simulink model "myproject_task"  (Simulink 3.00)
libraries: mathlib x17, inoutlib x13

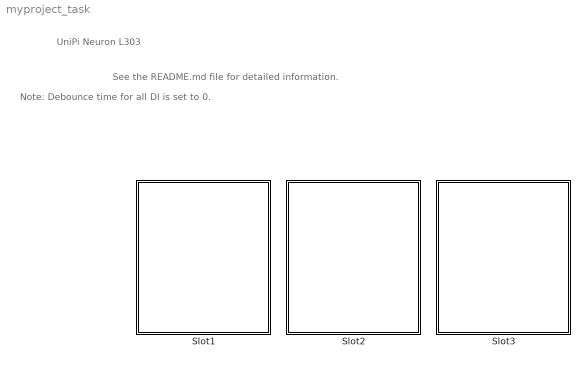
== system myproject_task ==
  note: See the README.md file for detailed information.
  note: UniPi Neuron L303
  note: Note: Debounce time for all DI is set to 0.
  Slot1 : Subsystem
      mask Type: REX sequence
  Slot2 : Subsystem
      mask Type: REX sequence
  Slot3 : Subsystem
      mask Type: REX sequence

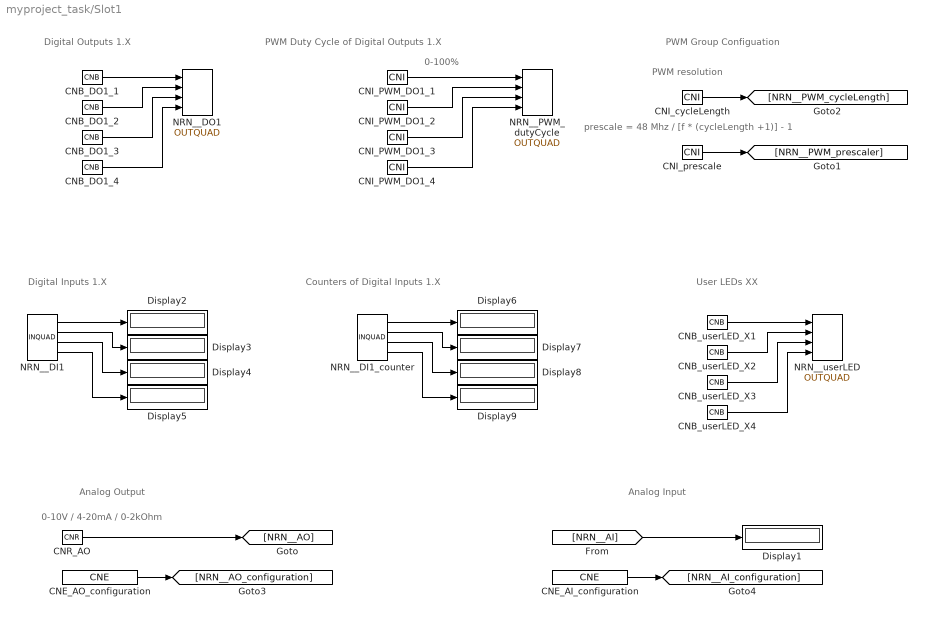
== system myproject_task/Slot1 ==
  note: 0-100%
  note: PWM resolution
  note: prescale = 48 Mhz / [f * (cycleLength +1)] - 1
  note: Digital Inputs 1.X
  note: Counters of Digital Inputs 1.X
  note: Digital Outputs 1.X
  note: User LEDs XX
  note: PWM Duty Cycle of Digital Outputs 1.X
  note: PWM Group Configuation
  note: 0-10V / 4-20mA / 0-2kOhm
  note: Analog Output
  note: Analog Input
  CNB_DO1_{1..4} (4 alike) : mathlib/CNB  YCN=off
  CNB_userLED_X{1..4} (4 alike) : mathlib/CNB  YCN=off
  CNE_AI_configuration : mathlib/CNE  yenum=0: Voltage 0-10V  pupstr=0: Voltage 0-10V|1: Current 0-20mA
  CNE_AO_configuration : mathlib/CNE  yenum=0: Voltage 0-10V  pupstr=0: Voltage 0-10V|1: Current 0-20mA|3: Resistance 0-2kOhm
  CNI_PWM_DO1_{1..4} (4 alike) : mathlib/CNI  icn=0
  CNI_cycleLength : mathlib/CNI  icn=1024
  CNI_prescale : mathlib/CNI  icn=467
  CNR_AO : mathlib/CNR  ycn=0
  Display{1..9} (9 alike) : Display
      Display1 settings: Format=short
      Display2 settings: Format=bin
      Display3 settings: Format=bin
      Display4 settings: Format=bin
      Display5 settings: Format=bin
      Display6 settings: Format=Best fit
      Display7 settings: Format=Best fit
      Display8 settings: Format=Best fit
      Display9 settings: Format=Best fit
  NRN__DI1 : inoutlib/INQUAD
  NRN__DI1_counter : inoutlib/INQUAD
  NRN__DO1 : inoutlib/OUTQUAD
  NRN__PWM_dutyCycle : inoutlib/OUTQUAD
  NRN__userLED : inoutlib/OUTQUAD
  wires:
  CNB_DO1_1/1 -> NRN__DO1/1
  CNB_DO1_2/1 -> NRN__DO1/2
  CNB_DO1_3/1 -> NRN__DO1/3
  CNB_DO1_4/1 -> NRN__DO1/4
  CNB_userLED_X1/1 -> NRN__userLED/1
  CNB_userLED_X2/1 -> NRN__userLED/2
  CNB_userLED_X3/1 -> NRN__userLED/3
  CNB_userLED_X4/1 -> NRN__userLED/4
  CNE_AI_configuration/1 -> [NRN__AI_configuration]
  CNE_AO_configuration/1 -> [NRN__AO_configuration]
  CNI_PWM_DO1_1/1 -> NRN__PWM_dutyCycle/1
  CNI_PWM_DO1_2/1 -> NRN__PWM_dutyCycle/2
  CNI_PWM_DO1_3/1 -> NRN__PWM_dutyCycle/3
  CNI_PWM_DO1_4/1 -> NRN__PWM_dutyCycle/4
  CNI_cycleLength/1 -> [NRN__PWM_cycleLength]
  CNI_prescale/1 -> [NRN__PWM_prescaler]
  CNR_AO/1 -> [NRN__AO]
  [NRN__AI] -> Display1/1
  NRN__DI1/1 -> Display2/1
  NRN__DI1/2 -> Display3/1
  NRN__DI1/3 -> Display4/1
  NRN__DI1/4 -> Display5/1
  NRN__DI1_counter/1 -> Display6/1
  NRN__DI1_counter/2 -> Display7/1
  NRN__DI1_counter/3 -> Display8/1
  NRN__DI1_counter/4 -> Display9/1

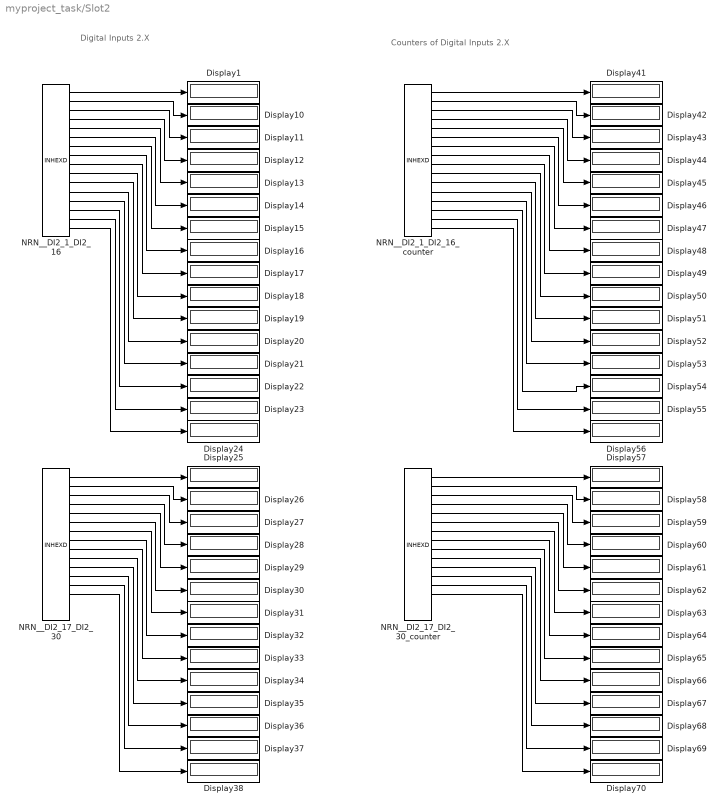
== system myproject_task/Slot2 ==
  note: Digital Inputs 2.X
  note: Counters of Digital Inputs 2.X
  Display{1,10..38,41..70} (60 alike) : Display
      Display1 settings: Format=bin
      Display10 settings: Format=bin
      Display11 settings: Format=bin
      Display12 settings: Format=bin
      Display13 settings: Format=bin
      Display14 settings: Format=bin
      Display15 settings: Format=bin
      Display16 settings: Format=bin
      Display17 settings: Format=bin
      Display18 settings: Format=bin
      Display19 settings: Format=bin
      Display20 settings: Format=bin
      Display21 settings: Format=bin
      Display22 settings: Format=bin
      Display23 settings: Format=bin
      Display24 settings: Format=bin
      Display25 settings: Format=bin
      Display26 settings: Format=bin
      Display27 settings: Format=bin
      Display28 settings: Format=bin
      Display29 settings: Format=bin
      Display30 settings: Format=bin
      Display31 settings: Format=bin
      Display32 settings: Format=bin
      Display33 settings: Format=bin
      Display34 settings: Format=bin
      Display35 settings: Format=bin
      Display36 settings: Format=bin
      Display37 settings: Format=bin
      Display38 settings: Format=bin
      Display41 settings: Format=Best fit
      Display42 settings: Format=Best fit
      Display43 settings: Format=Best fit
      Display44 settings: Format=Best fit
      Display45 settings: Format=Best fit
      Display46 settings: Format=Best fit
      Display47 settings: Format=Best fit
      Display48 settings: Format=Best fit
      Display49 settings: Format=Best fit
      Display50 settings: Format=Best fit
      Display51 settings: Format=Best fit
      Display52 settings: Format=Best fit
      Display53 settings: Format=Best fit
      Display54 settings: Format=Best fit
      Display55 settings: Format=Best fit
      Display56 settings: Format=Best fit
      Display57 settings: Format=Best fit
      Display58 settings: Format=Best fit
      Display59 settings: Format=Best fit
      Display60 settings: Format=Best fit
      Display61 settings: Format=Best fit
      Display62 settings: Format=Best fit
      Display63 settings: Format=Best fit
      Display64 settings: Format=Best fit
      Display65 settings: Format=Best fit
      Display66 settings: Format=Best fit
      Display67 settings: Format=Best fit
      Display68 settings: Format=Best fit
      Display69 settings: Format=Best fit
      Display70 settings: Format=Best fit
  NRN__DI2_17_DI2_30 : inoutlib/INHEXD
  NRN__DI2_17_DI2_30_counter : inoutlib/INHEXD
  NRN__DI2_1_DI2_16 : inoutlib/INHEXD
  NRN__DI2_1_DI2_16_counter : inoutlib/INHEXD
  wires:
  NRN__DI2_17_DI2_30/1 -> Display25/1
  NRN__DI2_17_DI2_30/2 -> Display26/1
  NRN__DI2_17_DI2_30/3 -> Display27/1
  NRN__DI2_17_DI2_30/4 -> Display28/1
  NRN__DI2_17_DI2_30/5 -> Display29/1
  NRN__DI2_17_DI2_30/6 -> Display30/1
  NRN__DI2_17_DI2_30/7 -> Display31/1
  NRN__DI2_17_DI2_30/8 -> Display32/1
  NRN__DI2_17_DI2_30/9 -> Display33/1
  NRN__DI2_17_DI2_30/10 -> Display34/1
  NRN__DI2_17_DI2_30/11 -> Display35/1
  NRN__DI2_17_DI2_30/12 -> Display36/1
  NRN__DI2_17_DI2_30/13 -> Display37/1
  NRN__DI2_17_DI2_30/14 -> Display38/1
  NRN__DI2_17_DI2_30_counter/1 -> Display57/1
  NRN__DI2_17_DI2_30_counter/2 -> Display58/1
  NRN__DI2_17_DI2_30_counter/3 -> Display59/1
  NRN__DI2_17_DI2_30_counter/4 -> Display60/1
  NRN__DI2_17_DI2_30_counter/5 -> Display61/1
  NRN__DI2_17_DI2_30_counter/6 -> Display62/1
  NRN__DI2_17_DI2_30_counter/7 -> Display63/1
  NRN__DI2_17_DI2_30_counter/8 -> Display64/1
  NRN__DI2_17_DI2_30_counter/9 -> Display65/1
  NRN__DI2_17_DI2_30_counter/10 -> Display66/1
  NRN__DI2_17_DI2_30_counter/11 -> Display67/1
  NRN__DI2_17_DI2_30_counter/12 -> Display68/1
  NRN__DI2_17_DI2_30_counter/13 -> Display69/1
  NRN__DI2_17_DI2_30_counter/14 -> Display70/1
  NRN__DI2_1_DI2_16/1 -> Display1/1
  NRN__DI2_1_DI2_16/2 -> Display10/1
  NRN__DI2_1_DI2_16/3 -> Display11/1
  NRN__DI2_1_DI2_16/4 -> Display12/1
  NRN__DI2_1_DI2_16/5 -> Display13/1
  NRN__DI2_1_DI2_16/6 -> Display14/1
  NRN__DI2_1_DI2_16/7 -> Display15/1
  NRN__DI2_1_DI2_16/8 -> Display16/1
  NRN__DI2_1_DI2_16/9 -> Display17/1
  NRN__DI2_1_DI2_16/10 -> Display18/1
  NRN__DI2_1_DI2_16/11 -> Display19/1
  NRN__DI2_1_DI2_16/12 -> Display20/1
  NRN__DI2_1_DI2_16/13 -> Display21/1
  NRN__DI2_1_DI2_16/14 -> Display22/1
  NRN__DI2_1_DI2_16/15 -> Display23/1
  NRN__DI2_1_DI2_16/16 -> Display24/1
  NRN__DI2_1_DI2_16_counter/1 -> Display41/1
  NRN__DI2_1_DI2_16_counter/2 -> Display42/1
  NRN__DI2_1_DI2_16_counter/3 -> Display43/1
  NRN__DI2_1_DI2_16_counter/4 -> Display44/1
  NRN__DI2_1_DI2_16_counter/5 -> Display45/1
  NRN__DI2_1_DI2_16_counter/6 -> Display46/1
  NRN__DI2_1_DI2_16_counter/7 -> Display47/1
  NRN__DI2_1_DI2_16_counter/8 -> Display48/1
  NRN__DI2_1_DI2_16_counter/9 -> Display49/1
  NRN__DI2_1_DI2_16_counter/10 -> Display50/1
  NRN__DI2_1_DI2_16_counter/11 -> Display51/1
  NRN__DI2_1_DI2_16_counter/12 -> Display52/1
  NRN__DI2_1_DI2_16_counter/13 -> Display53/1
  NRN__DI2_1_DI2_16_counter/14 -> Display54/1
  NRN__DI2_1_DI2_16_counter/15 -> Display55/1
  NRN__DI2_1_DI2_16_counter/16 -> Display56/1

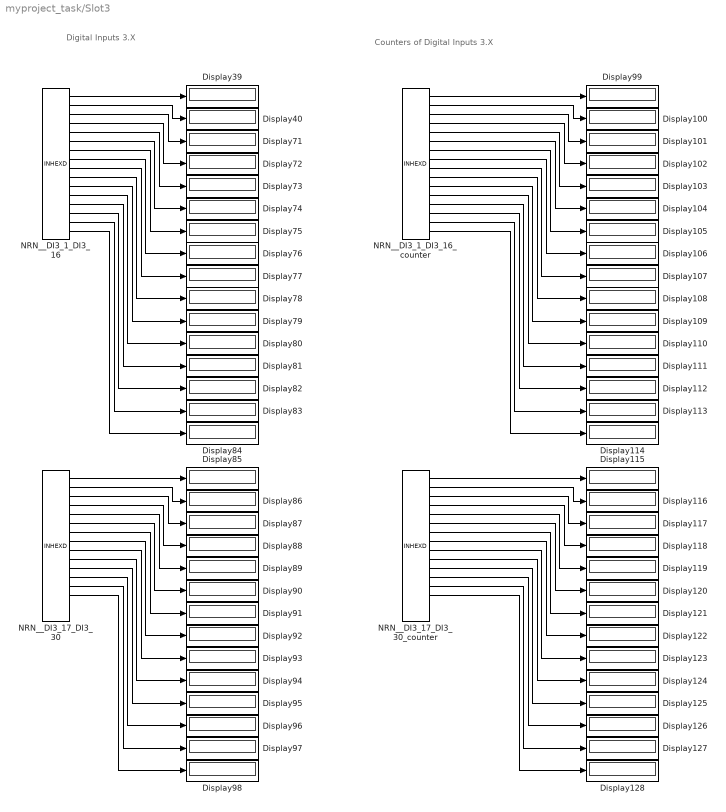
== system myproject_task/Slot3 ==
  note: Digital Inputs 3.X
  note: Counters of Digital Inputs 3.X
  Display{39..40,71..128} (60 alike) : Display
      Display100 settings: Format=Best fit
      Display101 settings: Format=Best fit
      Display102 settings: Format=Best fit
      Display103 settings: Format=Best fit
      Display104 settings: Format=Best fit
      Display105 settings: Format=Best fit
      Display106 settings: Format=Best fit
      Display107 settings: Format=Best fit
      Display108 settings: Format=Best fit
      Display109 settings: Format=Best fit
      Display110 settings: Format=Best fit
      Display111 settings: Format=Best fit
      Display112 settings: Format=Best fit
      Display113 settings: Format=Best fit
      Display114 settings: Format=Best fit
      Display115 settings: Format=Best fit
      Display116 settings: Format=Best fit
      Display117 settings: Format=Best fit
      Display118 settings: Format=Best fit
      Display119 settings: Format=Best fit
      Display120 settings: Format=Best fit
      Display121 settings: Format=Best fit
      Display122 settings: Format=Best fit
      Display123 settings: Format=Best fit
      Display124 settings: Format=Best fit
      Display125 settings: Format=Best fit
      Display126 settings: Format=Best fit
      Display127 settings: Format=Best fit
      Display128 settings: Format=Best fit
      Display39 settings: Format=bin
      Display40 settings: Format=bin
      Display71 settings: Format=bin
      Display72 settings: Format=bin
      Display73 settings: Format=bin
      Display74 settings: Format=bin
      Display75 settings: Format=bin
      Display76 settings: Format=bin
      Display77 settings: Format=bin
      Display78 settings: Format=bin
      Display79 settings: Format=bin
      Display80 settings: Format=bin
      Display81 settings: Format=bin
      Display82 settings: Format=bin
      Display83 settings: Format=bin
      Display84 settings: Format=bin
      Display85 settings: Format=bin
      Display86 settings: Format=bin
      Display87 settings: Format=bin
      Display88 settings: Format=bin
      Display89 settings: Format=bin
      Display90 settings: Format=bin
      Display91 settings: Format=bin
      Display92 settings: Format=bin
      Display93 settings: Format=bin
      Display94 settings: Format=bin
      Display95 settings: Format=bin
      Display96 settings: Format=bin
      Display97 settings: Format=bin
      Display98 settings: Format=bin
      Display99 settings: Format=Best fit
  NRN__DI3_17_DI3_30 : inoutlib/INHEXD
  NRN__DI3_17_DI3_30_counter : inoutlib/INHEXD
  NRN__DI3_1_DI3_16 : inoutlib/INHEXD
  NRN__DI3_1_DI3_16_counter : inoutlib/INHEXD
  wires:
  NRN__DI3_17_DI3_30/1 -> Display85/1
  NRN__DI3_17_DI3_30/2 -> Display86/1
  NRN__DI3_17_DI3_30/3 -> Display87/1
  NRN__DI3_17_DI3_30/4 -> Display88/1
  NRN__DI3_17_DI3_30/5 -> Display89/1
  NRN__DI3_17_DI3_30/6 -> Display90/1
  NRN__DI3_17_DI3_30/7 -> Display91/1
  NRN__DI3_17_DI3_30/8 -> Display92/1
  NRN__DI3_17_DI3_30/9 -> Display93/1
  NRN__DI3_17_DI3_30/10 -> Display94/1
  NRN__DI3_17_DI3_30/11 -> Display95/1
  NRN__DI3_17_DI3_30/12 -> Display96/1
  NRN__DI3_17_DI3_30/13 -> Display97/1
  NRN__DI3_17_DI3_30/14 -> Display98/1
  NRN__DI3_17_DI3_30_counter/1 -> Display115/1
  NRN__DI3_17_DI3_30_counter/2 -> Display116/1
  NRN__DI3_17_DI3_30_counter/3 -> Display117/1
  NRN__DI3_17_DI3_30_counter/4 -> Display118/1
  NRN__DI3_17_DI3_30_counter/5 -> Display119/1
  NRN__DI3_17_DI3_30_counter/6 -> Display120/1
  NRN__DI3_17_DI3_30_counter/7 -> Display121/1
  NRN__DI3_17_DI3_30_counter/8 -> Display122/1
  NRN__DI3_17_DI3_30_counter/9 -> Display123/1
  NRN__DI3_17_DI3_30_counter/10 -> Display124/1
  NRN__DI3_17_DI3_30_counter/11 -> Display125/1
  NRN__DI3_17_DI3_30_counter/12 -> Display126/1
  NRN__DI3_17_DI3_30_counter/13 -> Display127/1
  NRN__DI3_17_DI3_30_counter/14 -> Display128/1
  NRN__DI3_1_DI3_16/1 -> Display39/1
  NRN__DI3_1_DI3_16/2 -> Display40/1
  NRN__DI3_1_DI3_16/3 -> Display71/1
  NRN__DI3_1_DI3_16/4 -> Display72/1
  NRN__DI3_1_DI3_16/5 -> Display73/1
  NRN__DI3_1_DI3_16/6 -> Display74/1
  NRN__DI3_1_DI3_16/7 -> Display75/1
  NRN__DI3_1_DI3_16/8 -> Display76/1
  NRN__DI3_1_DI3_16/9 -> Display77/1
  NRN__DI3_1_DI3_16/10 -> Display78/1
  NRN__DI3_1_DI3_16/11 -> Display79/1
  NRN__DI3_1_DI3_16/12 -> Display80/1
  NRN__DI3_1_DI3_16/13 -> Display81/1
  NRN__DI3_1_DI3_16/14 -> Display82/1
  NRN__DI3_1_DI3_16/15 -> Display83/1
  NRN__DI3_1_DI3_16/16 -> Display84/1
  NRN__DI3_1_DI3_16_counter/1 -> Display99/1
  NRN__DI3_1_DI3_16_counter/2 -> Display100/1
  NRN__DI3_1_DI3_16_counter/3 -> Display101/1
  NRN__DI3_1_DI3_16_counter/4 -> Display102/1
  NRN__DI3_1_DI3_16_counter/5 -> Display103/1
  NRN__DI3_1_DI3_16_counter/6 -> Display104/1
  NRN__DI3_1_DI3_16_counter/7 -> Display105/1
  NRN__DI3_1_DI3_16_counter/8 -> Display106/1
  NRN__DI3_1_DI3_16_counter/9 -> Display107/1
  NRN__DI3_1_DI3_16_counter/10 -> Display108/1
  NRN__DI3_1_DI3_16_counter/11 -> Display109/1
  NRN__DI3_1_DI3_16_counter/12 -> Display110/1
  NRN__DI3_1_DI3_16_counter/13 -> Display111/1
  NRN__DI3_1_DI3_16_counter/14 -> Display112/1
  NRN__DI3_1_DI3_16_counter/15 -> Display113/1
  NRN__DI3_1_DI3_16_counter/16 -> Display114/1
